simulink model "lqr_daolibai_1"  (R2015b)
settings: Solver=VariableStepAuto  StartTime=0.0  StopTime=10.0  RelTol=1e-3
values from neighbouring files (symbols this model uses):
  Ac = [(A-B*K)]    [lqr_daolibai.m]    (also in lqr_daolibai2.m = A - B*K)
  C = [ 1 0 0 0;    0 0 1 0]    [lqr_daolibai.m]    (also in lqr_daolibai2.m = [0 0 1 0])
  D = [ 0 0 ]'    [lqr_daolibai.m]    (also in lqr_daolibai2.m = 0)
settings Model: Creator=Administrator  LastModifiedBy=Administrator

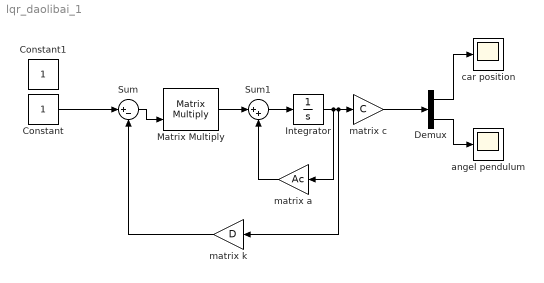
== system lqr_daolibai_1 ==
  Constant : Constant
  Constant1 : Constant
  Demux : Demux  Outputs=2
  Integrator : Integrator
  Matrix Multiply : Product  Multiplication=Matrix(*)
  Sum : Sum  Inputs=|+-
  Sum1 : Sum  Inputs=|++
  angel pendulum : Scope
  car position : Scope
  matrix a : Gain  Gain=Ac
  matrix c : Gain  Gain=C
  matrix k : Gain  Gain=D
  wires:
  Constant/1 -> Sum/1
  Matrix Multiply/1 -> Sum1/1
  Sum1/1 -> Integrator/1
  matrix c/1 -> Demux/1
  Demux/1 -> car position/1
  Demux/2 -> angel pendulum/1
  Integrator/1 -> matrix a/1, matrix k/1, matrix c/1
  matrix a/1 -> Sum1/2
  matrix k/1 -> Sum/2
  Sum/1 -> Matrix Multiply/2
